simulink library "lib_TCML"  (R2015a)
(part 2 of 7)

      | MSK_SEC_Enables_TMATS('E_TempDependence_Rotor_M',[58 59],'en')
      mask Callback v_TempDependence_Rotor_M:
      | MSK_SEC_Enables_TMATS('v_TempDependence_Rotor_M',61,'dis')
      | MSK_SEC_Enables_TMATS('v_TempDependence_Rotor_M',[62 63],'en')
      mask Callback k_TempDependence_Case_M:
      | MSK_SEC_Enables_TMATS('k_TempDependence_Case_M',69,'dis')
      | MSK_SEC_Enables_TMATS('k_TempDependence_Case_M',[70 71],'en')
      mask Callback h_Const_Case_In_M:
      | if length(get_param(gcb,'h_Const_Case_In_M')) == 2 %on
      |     set_param(gcb,'h_Eqn_Case_In_M','off');
      |     set_param(gcb,'h_Data_Case_In_M','off');
      |     MSK_SEC_Enables2_TMATS('h_Const_Case_In_M',75,'en')
      |     MSK_SEC_Enables2_TMATS('h_Const_Case_In_M',[76 77 78 79 80 81],'dis')
      | end
      mask Callback h_Eqn_Case_In_M:
      | if length(get_param(gcb,'h_Eqn_Case_In_M')) == 2 %on
      |     set_param(gcb,'h_Const_Case_In_M','off');
      |     set_param(gcb,'h_Data_Case_In_M','off');
      |     MSK_SEC_Enables2_TMATS('h_Eqn_Case_In_M',[76 77 78],'en')
      |     MSK_SEC_Enables2_TMATS('h_Eqn_Case_In_M',[75 79 80 81],'dis')
      | end
      mask Callback h_Data_Case_In_M:
      | if length(get_param(gcb,'h_Data_Case_In_M')) == 2 %on
      |     set_param(gcb,'h_Eqn_Case_In_M','off');
      |     set_param(gcb,'h_Const_Case_In_M','off');
      |     MSK_SEC_Enables2_TMATS('h_Data_Case_In_M',[75 76],'dis')
      |     MSK_SEC_Enables2_TMATS('h_Data_Case_In_M',[77 78 79 80 81],'en')
      | end
      mask Callback h_Const_Case_Out_M:
      | if length(get_param(gcb,'h_Const_Case_Out_M')) == 2 %on
      |     set_param(gcb,'h_Eqn_Case_Out_M','off');
      |     set_param(gcb,'h_Data_Case_Out_M','off');
      |     MSK_SEC_Enables2_TMATS('h_Const_Case_Out_M',85,'en')
      |     MSK_SEC_Enables2_TMATS('h_Const_Case_Out_M',[86 87 88 89 90 91],'dis')
      | end
      mask Callback h_Eqn_Case_Out_M:
      | if length(get_param(gcb,'h_Eqn_Case_Out_M')) == 2 %on
      |     set_param(gcb,'h_Const_Case_Out_M','off');
      |     set_param(gcb,'h_Data_Case_Out_M','off');
      |     MSK_SEC_Enables2_TMATS('h_Eqn_Case_Out_M',[86 87 88],'en')
      |     MSK_SEC_Enables2_TMATS('h_Eqn_Case_Out_M',[85 89 90 91],'dis')
      | end
      mask Callback h_Data_Case_Out_M:
      | if length(get_param(gcb,'h_Data_Case_Out_M')) == 2 %on
      |     set_param(gcb,'h_Eqn_Case_Out_M','off');
      |     set_param(gcb,'h_Const_Case_Out_M','off');
      |     MSK_SEC_Enables2_TMATS('h_Data_Case_Out_M',[85 86],'dis')
      |     MSK_SEC_Enables2_TMATS('h_Data_Case_Out_M',[87 88 89 90 91],'en')
      | end
      mask Callback alpha_TempDependence_Case_M:
      | MSK_SEC_Enables_TMATS('alpha_TempDependence_Case_M',95,'dis')
      | MSK_SEC_Enables_TMATS('alpha_TempDependence_Case_M',[96 97],'en')
      mask DialogControl Container36 Prompt: Model Selection
      mask DialogControl Container33 Prompt: Thermal Expansion Coefficient
      mask DialogControl Container37 Prompt: Young's Modulus
      mask DialogControl Container25 Prompt: Material properties
      mask DialogControl Container26 Prompt: Thermal conductivity
      mask DialogControl Container38 Prompt: Thermal expansion coefficient
      mask DialogControl Container40 Prompt: Young's Modulus
      mask DialogControl Container41 Prompt: Poisson's Ratio
      mask DialogControl Container51 Prompt: Material Properties
      mask DialogControl Container52 Prompt: Thermal conductivity
      mask DialogControl Container63 Prompt: Thermal Expansion Coefficient
  Tip Clearance Effect on Performance : Subsystem  mask(TCML - Tip Clearance Effect on Performance Library Block){L_Shroud_M=1/12, DegGap_M=0, NomConfig_M=on}
      mask prompts: L_Shroud_M "L_Shroud_M - Shroud offset (distance between the inner surface of the shroud and the inner surface of the casing) [ft]"; DegGap_M "DegGap_M - Degradation gap (off-nominal increase in the tip clearance gap due to degradation) [mils]"; NomConfig_M "NomConfig_M - Nominal configuration option (unchecked - nominal configuration is represented inside the "Dynamic Tip Clearance Block", checked - otherwise)"
      mask help:
      | This block produces an estimate of the tip clearance impact on the efficiency of the turbomachinery component. It accepts the output structure from a "Dynamic Tip Clearance" block, the displacement of a tip clearance actuator (if one exists), and a performance impact coefficient (described in the help menu) along with the constant parameters of the degradation gap (see below) and shroud offset distance (see below) to determine the factor by which the efficiency is impacted. The factor can be multiplied by the component efficiency scaler in an engine simulation to achieve the appropriate component efficiency. Therefore, the output is refered to as the efficiency scaler coefficient. The NomConfig_M parameter is 0 (unchecked) by default which assumes that the turbine configuration defined in the "Dynamic Tip Clearance" block (material, dimensions, etc.) represent the nominal configuration that correlates to the nominal tip clearance and component performance. If this is not true then the NomConfig_M checkbox can be checked and a new inport will appear that asks for the nominal tip clearance. This nominal tip clearance value will override the nominal tip clearance produced by the "Dynamic Tip Clearance" block. Instead the nominal tip clearance should be supplied by a "Steady-State Tip Clearance" block whose inputs are the same as the "Dynamic Tip Clearance" block but whose parameters are consistent with the nominal turbine configuration.
      |
      | Refer to the help menu for more information about this block.
      mask init:
      | % Inport Numbers
      | n = 4; %first inport number
      | 
      | % Core Mass Flow Rate Inport
      | if NomConfig_M == 1
      |     if strcmp(get_param([gcb '/Nominal Config. TC (mils)'],'BlockType'),'Constant')
      |         MSK_ReplaceBlock_TMATS([gcb '/Nominal Config. TC (mils)'],'built-in/Inport');
      |     end
      |     set_param([gcb '/Nominal Config. TC (mils)'],'Port',num2str(n));
      | else
      |     if strcmp(get_param([gcb '/Nominal Config. TC (mils)'],'BlockType'),'Inport')
      |         MSK_ReplaceBlock_TMATS([gcb '/Nominal Config. TC (mils)'],'built-in/Constant');
      |         set_param([gcb '/Nominal Config. TC (mils)'],'Value','1');
      |     end
      | end
      mask Help: web(which('TipClearEffPerf.html'),'-helpbrowser')
